simulink subsystem "mission4"  (R2024a)
settings: Solver=VariableStepAuto  StartTime=0.0  StopTime=10.0  RelTol=1e-3
settings Model: Creator=User  LastModifiedBy=User

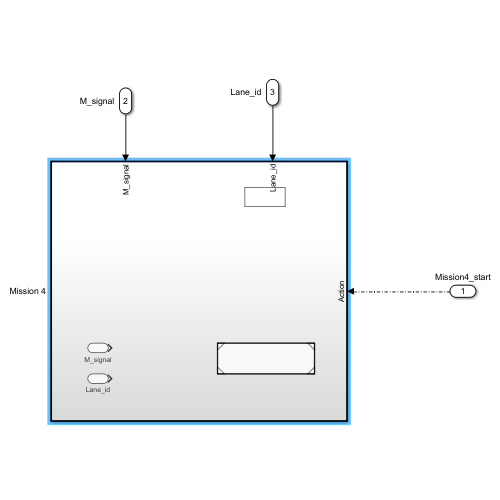
[thumbnail: Simulink's stored preview of the top-level diagram]
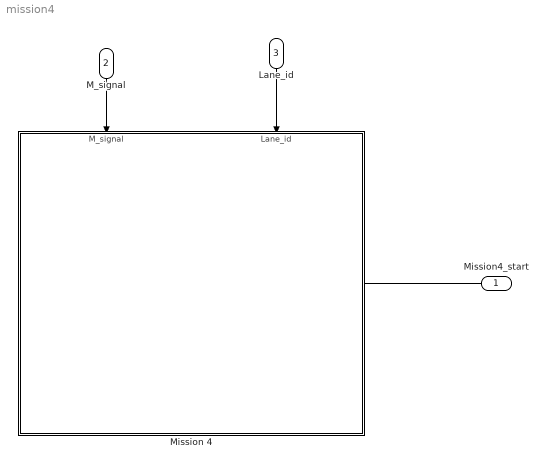
== system mission4 ==
  Mission4_start : Inport
  M_signal : Inport  Port=2
  Lane_id : Inport  Port=3
  Mission 4 : Subsystem  TreatAsAtomicUnit=on
  wires:
  M_signal/1 -> Mission 4/1(M_signal)
  Lane_id/1 -> Mission 4/2(Lane_id)
  Mission4_start/1 -> Mission 4/Action

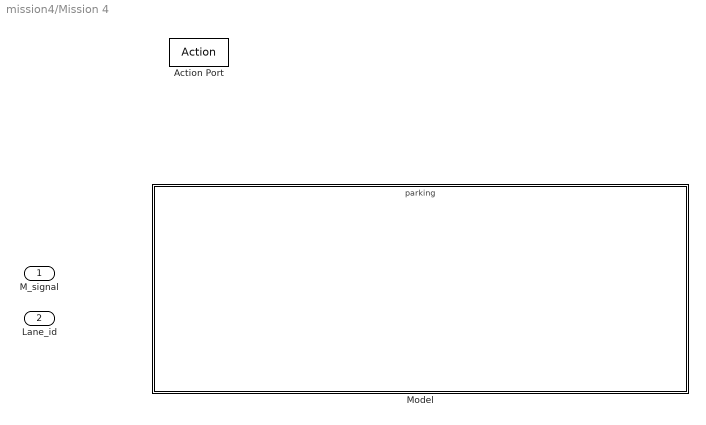
== system mission4/Mission 4 ==
  M_signal : Inport
  Lane_id : Inport  Port=2
  Action Port : ActionPort
  Model : ModelReference  ModelNameDialog=parking.slx  SimulationMode=Normal  ModelReferenceVersion=1.3
